simulink library "PowerMeter"  (R2018b)
settings: Solver=ode45  StartTime=0.0  StopTime=10.0  RelTol=1e-3  EnableMultiTasking=on
libraries: carnot x1
settings Model: Creator=drhf  LastModifiedBy=P41573
settings DataIOCC: LimitDataPoints=on  SaveFormat=Array  SignalLoggingSaveFormat=ModelDataLogs
settings OptimizationCC: ExpressionDepthLimit=2147483647  LifeSpan=inf
settings DebuggingCC: UnderspecifiedInitializationDetection=Classic  MergeDetectMultiDrivingBlocksExec=none  SolverPrmCheckMsg=warning  FcnCallInpInsideContextMsg=warning  StateNameClashWarn=warning  SFUnexpectedBacktrackingDiag=warning  SFNoUnconditionalDefaultTransitionDiag=warning  SFExecutionAtInitializationDiag=none
settings HardwareCC: ProdBitPerPointer=32  ProdBitPerSizeT=32  ProdBitPerPtrDiffT=32  ProdLargestAtomicFloat=None  ProdIntDivRoundTo=Undefined  ProdEndianess=Unspecified  ProdWordSize=32  ProdHWDeviceType=32-bit Generic
settings ModelReferenceCC: PropagateSignalLabelsOutOfModel=off
settings SFSimCC: SimUseLocalCustomCode=off
settings RTWCC: RTWUseLocalCustomCode=off
settings CodeAppCC: StateflowObjectComments=on
settings GRTTargetCC: TargetLangStandard=C89/C90 (ANSI)  GeneratePreprocessorConditionals=Disable all  CombineOutputUpdateFcns=off  GRTInterface=on
settings ConfigComp: CovMetricSettings=dw  CovHtmlReporting=on  CovSaveCumulativeToWorkspaceVar=on  CovSaveSingleToWorkspaceVar=on  CovExternalEMLEnable=off

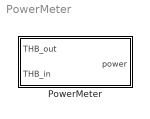
== system PowerMeter ==
  PowerMeter : Subsystem  mask(power meter){}
      mask help:
      | Calculates the power of a fluid flow between inlet and outlet of components characterized by the THB.
      | Qdot = mdot * cp(Tmean) * (Tout - Tin)
      | Tmean = (Tin+Tout)/2
      mask Help: web(fullfile(path_carnot('help'),'PowerMeter.html'),'-helpbrowser')

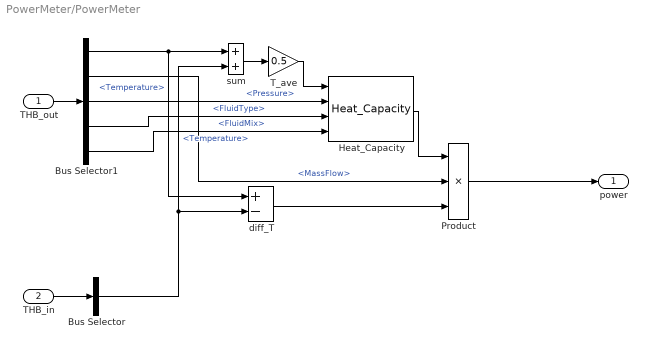
== system PowerMeter/PowerMeter ==
  THB_out : Inport
  THB_in : Inport  Port=2
  Bus Selector : BusSelector  OutputSignals=Temperature
  Bus Selector1 : BusSelector  OutputSignals=Temperature,MassFlow,Pressure,FluidType,FluidMix
  Heat_Capacity : carnot/Basic/Material_Properties/Heat_Capacity  VariantControl=CarlibClassic  INPUTARGUMENTS=state variables (classic)  DEBUGLEVEL=DEBUGLEVEL  MAXTOTALWARNINGS=inf  MAXCONSECUTIVEWARNINGS=inf  WRITETOFILE=0  FILENAME='errors.txt'
      settings: SourceProductName=Carnot
  Product : Product  Inputs=***  SaturateOnIntegerOverflow=on  InputSameDT=on  OutDataTypeStr=Inherit: Same as first input
  T_ave : Gain  Gain=0.5  SaturateOnIntegerOverflow=on  OutDataTypeStr=Inherit: Same as input  ParamDataTypeStr=Inherit: Same as input
  diff_T : Sum  Inputs=+-  SaturateOnIntegerOverflow=on  InputSameDT=on  OutDataTypeStr=Inherit: Same as first input
  sum : Sum  SaturateOnIntegerOverflow=on  InputSameDT=on  OutDataTypeStr=Inherit: Same as first input
  power : Outport
  wires:
  THB_out/1 -> Bus Selector1/1
  Bus Selector1/3 -> Heat_Capacity/2  "<Pressure>"
  T_ave/1 -> Heat_Capacity/1
  sum/1 -> T_ave/1
  Bus Selector/1 -> sum/2, diff_T/2  "<Temperature>"
  THB_in/1 -> Bus Selector/1
  diff_T/1 -> Product/3
  Bus Selector1/2 -> Product/2  "<MassFlow>"
  Product/1 -> power/1
  Heat_Capacity/1 -> Product/1
  Bus Selector1/5 -> Heat_Capacity/4  "<FluidMix>"
  Bus Selector1/4 -> Heat_Capacity/3  "<FluidType>"
  Bus Selector1/1 -> sum/1, diff_T/1  "<Temperature>"
